simulink model "task11_8"  (R2021a)
settings: Solver=VariableStepAuto  StartTime=0.0  StopTime=10.0  RelTol=1e-3
libraries: simulink x1
settings Model: Creator=reemb  LastModifiedBy=reemb

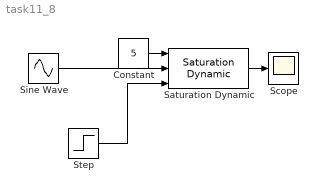
== system task11_8 ==
  Constant : Constant  Value=5
  Saturation Dynamic : simulink/Discontinuities/Saturation Dynamic  OutMin=[]  OutMax=[]  OutDataTypeStr=Inherit: Same as second input  OutDataType=fixdt(1, 16)  OutScaling=2^-10  RndMeth=Round  DoSatur=off
  Scope : Scope
  Sine Wave : Sin  Amplitude=10  SampleTime=0
  Step : Step  Time=5  Before=-10  After=0  SampleTime=0
  wires:
  Sine Wave/1 -> Saturation Dynamic/2
  Step/1 -> Saturation Dynamic/3
  Saturation Dynamic/1 -> Scope/1
  Constant/1 -> Saturation Dynamic/1
